simulink model "nonsim"  (Simulink 7.0)
settings: Solver=ode45  StartTime=0.0  StopTime=150.0  RelTol=1e-3
values from neighbouring files (symbols this model uses):
  a = [f, 0*f ... (first row only)    [fig10_18.m]    (also in fig10_19.m; fig10_20.m; fig10_21.m; fig10_22.m)
  N = 1.00    (= 1)    [f_tos.m]
  r = rlocus(Aol,Bol,Col,Dol,k5)    [fig10_15.m]    (also in fig10_18.m = [0*g;1]; fig10_19.m = [0*g;1]; fig10_20.m = [0*g;1]; fig10_21.m = [0*g;1])
undefined symbols (not defined in the file or in its folder): den, df, nf, num
settings Model: Creator=abbas  LastModifiedBy=abbas  ExtModeTrigMode=oneshot  ExtModeArmWhenConnect=off
settings DataIOCC: LimitDataPoints=off
settings OptimizationCC: BlockReduction=off  BooleanDataType=off
settings DebuggingCC: SaveWithParameterizedLinksMsg=none  SignalResolutionControl=TryResolveAllWithWarning  SolverPrmCheckMsg=none  MultiTaskDSMMsg=warning  MultiTaskCondExecSysMsg=none  StrictBusMsg=None
settings HardwareCC: TargetUnknown=on
settings RTWCC: IncludeERTFirstTime=on
settings STFCustomTargetCC: GenFloatMathFcnCalls=ANSI_C  ModelReferenceCompliant=off  SystemTargetFile=grt.tlc

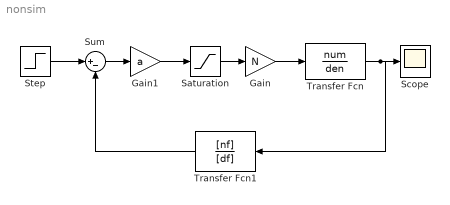
== system nonsim ==
  Gain : Gain  Gain=N  SaturateOnIntegerOverflow=on
  Gain1 : Gain  Gain=a  SaturateOnIntegerOverflow=on
  Saturation : Saturate  UpperLimit=1  LowerLimit=-1
  Scope : Scope
      settings: SaveName=yn  DataFormat=Array
  Step : Step  Time=.1  After=r  SampleTime=0.01
  Sum : Sum  Inputs=|+-  SaturateOnIntegerOverflow=on  InputSameDT=on
  Transfer Fcn : TransferFcn  Numerator=num  Denominator=den
  Transfer Fcn1 : TransferFcn  Orientation=left  Numerator=[nf]  Denominator=[df]
  wires:
  Step/1 -> Sum/1
  Gain1/1 -> Saturation/1
  Sum/1 -> Gain1/1
  Saturation/1 -> Gain/1
  Gain/1 -> Transfer Fcn/1
  Transfer Fcn/1 -> Scope/1, Transfer Fcn1/1
  Transfer Fcn1/1 -> Sum/2
